simulink model "hexa_quaternion_observer_ANSFT"  (R2023a)
settings: Solver=ode1  StartTime=0.0  StopTime=5  FixedStep=0.01  RelTol=1e-3
undefined symbols (not defined in the file or in its folder): F, Light, MIL
libraries: dspsrcs4 x9, aerolibutil x8, sharedtransform x8, simulink x5, matrix_library x3, sharedutil x3, simulink_extras x3, robotcorelib x1, aerolibwind2 x1, uavutilslib x1
(part 1 of 2)
settings Model: Creator=adan  LastModifiedBy=adan

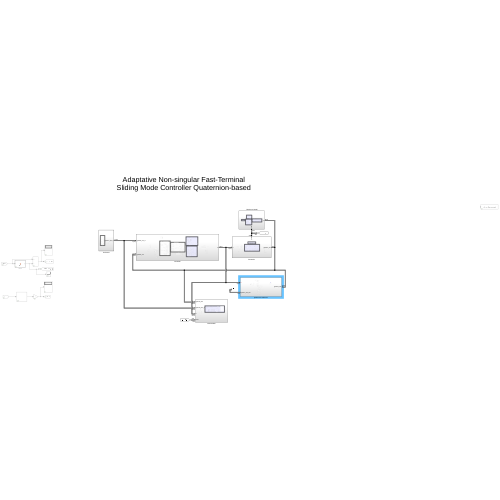
[thumbnail: Simulink's stored preview of the top-level diagram]
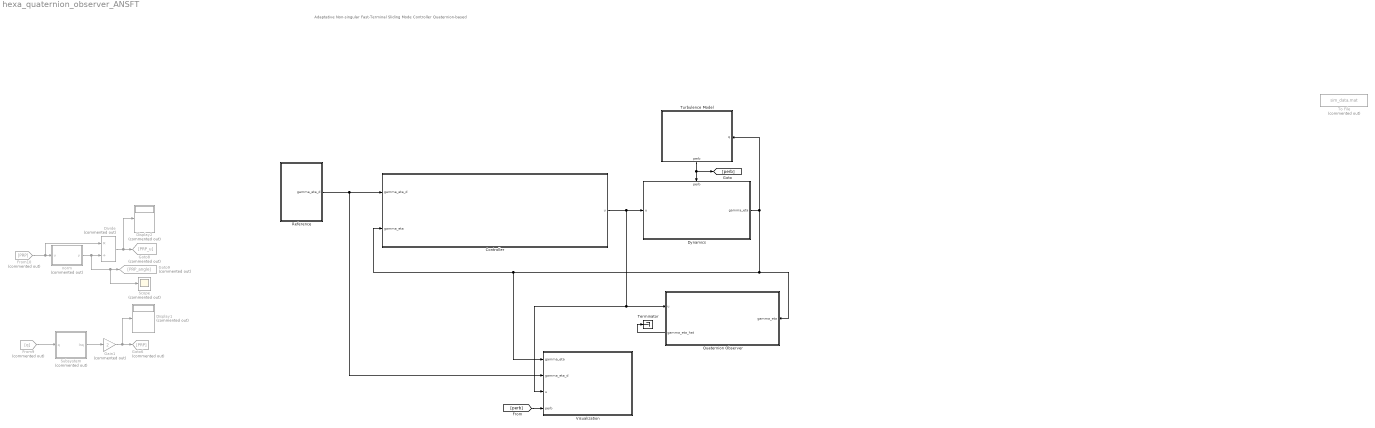
== system hexa_quaternion_observer_ANSFT ==
  note: Adaptative Non-singular Fast-Terminal Sliding Mode Controller Quaternion-based
  Controller : Subsystem
  Display1 : Display  Commented=on
  Display2 : Display  Commented=on
  Divide : Product  Commented=on  Inputs=*/
  Dynamics : Subsystem
      settings: PortSchema="{\"entries\":[{\"content\":{\"sides\":[{\"content\":{\"connectorIds\":[\"In1\"]},\"type\":\"ConnectorPlacement.EquallySpacedRectSide\",\"uuid\":\"7633f0a6-af79-48e6-9c86-d26739dbb2cd\"},{\"content\":{\"connectorIds\":[\"Out1\"],\"side\":\"RIGHT\"},\"type\":\"ConnectorPlacement.EquallySpacedRectSide\",\"uuid\":\"142aa0cc-a83e-43d8-8343-5180a7a0e227\"},{\"content\":{\"connectorIds\":[\"In2\"],\"side\":\"TOP\"},\"type\":\"ConnectorPlacement.EquallySpacedRectSide\",\"uuid\":\"a56720e4-09a6-4924-9ad2-7923d5a06f98\"}]},\"type\":\"ConnectorPlacement.EquallySpacedConnector\",\"uuid\":\"53d234f7-5315-4b90-bf85-0e64865b94b3\"}],\"packageUris\":[\"http://schema.mathworks.com/mf0/Connector/R2020b\"],\"version\":\"1.0\"}"
  From10 : From  Commented=on  GotoTag=PRP
  From9 : From  Commented=on  GotoTag=q
  Gain1 : Gain  Commented=on  Gain=2
  Goto6 : Goto  Commented=on  GotoTag=PRP
  Goto8 : Goto  Commented=on  GotoTag=PRP_u
  Goto9 : Goto  Commented=on  GotoTag=PRP_angle
  Quaternion Observer : Subsystem
      settings: PortSchema="{\"entries\":[{\"content\":{\"sides\":[{\"content\":{\"connectorIds\":[\"In1\"]},\"type\":\"ConnectorPlacement.EquallySpacedRectSide\",\"uuid\":\"43dabb6c-5b7b-4e74-9fbb-877aa2e7320c\"},{\"content\":{\"connectorIds\":[\"In2\",\"Out1\"],\"side\":\"RIGHT\"},\"type\":\"ConnectorPlacement.EquallySpacedRectSide\",\"uuid\":\"9ed47776-94ef-4325-8624-b198cf9ddeb6\"},{\"content\":{\"side\":\"TOP\"},\"type\":\"ConnectorPlacement.EquallySpacedRectSide\",\"uuid\":\"b1e3d92d-3c8b-4698-8faf-48c27cfda7a8\"}]},\"type\":\"ConnectorPlacement.EquallySpacedConnector\",\"uuid\":\"a3be4682-1c06-4ed6-a307-3a935f166e03\"}],\"packageUris\":[\"http://schema.mathworks.com/mf0/Connector/R2020b\"],\"version\":\"1.0\"}"
  Reference : Subsystem
  Scope : Scope  Commented=on
  Subsystem : Subsystem  Commented=on
  Terminator : Terminator
  To File : ToFile  Commented=on  Filename=sim_data.mat  MatrixName=out
  Turbulence Model : Subsystem
      settings: PortSchema="{\"entries\":[{\"content\":{\"sides\":[{\"content\":{},\"type\":\"ConnectorPlacement.EquallySpacedRectSide\",\"uuid\":\"1a11629b-61d3-4a8e-8df8-8509e014e579\"},{\"content\":{\"connectorIds\":[\"In1\"],\"side\":\"RIGHT\"},\"type\":\"ConnectorPlacement.EquallySpacedRectSide\",\"uuid\":\"4b15c564-9714-4da5-9436-a08c0d95800f\"},{\"content\":{\"side\":\"TOP\"},\"type\":\"ConnectorPlacement.EquallySpacedRectSide\",\"uuid\":\"dd21b825-2def-4360-b27b-b8c6f475bfab\"},{\"content\":{\"connectorIds\":[\"Out1\"],\"side\":\"BOTTOM\"},\"type\":\"ConnectorPlacement.EquallySpacedRectSide\",\"uuid\":\"594b79ea-4a45-43b1-b592-64a34d0135fb\"}]},\"type\":\"ConnectorPlacement.EquallySpacedConnector\",\"uuid\":\"4c6e67eb-825c-4dd0-a48b-2afa68ae74f5\"}],\"packageUris\":[\"http://schema.mathworks.com/mf0/Connector/R2020b\"],\"version\":\"1.0\"}"
  Visualization : Subsystem
  norm : MATLAB Function  Commented=on  TreatAsAtomicUnit=on
  wires:
  From9/1 -> Subsystem/1(q)
  Subsystem/1(lnq) -> Gain1/1
  Gain1/1 -> Display1/1, Goto6/1
  From10/1 -> norm/1(u), Divide/1
  norm/1(y) -> Scope/1, Goto9/1, Divide/2
  Divide/1 -> Goto8/1, Display2/1
  Reference/1(gamma_eta_d) -> Controller/1(gamma_eta_d), Visualization/2(gamma_eta_d)
  Controller/1(u) -> Quaternion Observer/2(u), Visualization/3(u), Dynamics/1(u)
  Dynamics/1(gamma_eta) -> Turbulence Model/1(q), Quaternion Observer/1(gamma_eta), Visualization/1(gamma_eta), Controller/2(gamma_eta)
  Turbulence Model/1(perb) -> [perb], Dynamics/2(perb)
  Quaternion Observer/1(gamma_eta_hat) -> Terminator/1
  [perb] -> Visualization/4(perb)

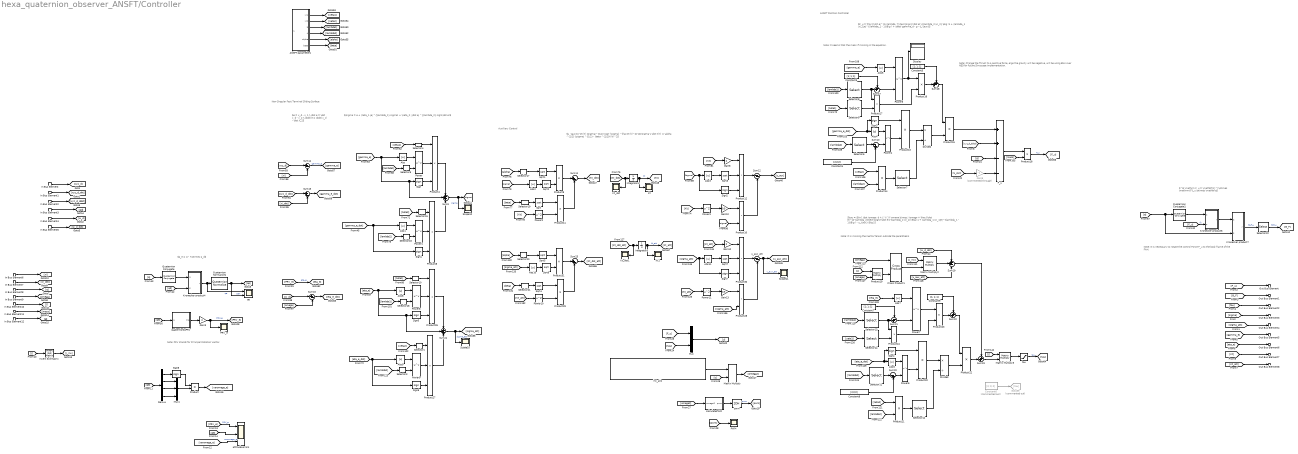
== system hexa_quaternion_observer_ANSFT/Controller ==
  note: $q_e = q^ *\otimes q_d$
  note: Non-Singular Fast Terminal Sliding Surface
  note: $\sigma = e + \zeta_1 |e| ^{\lambda_1} sign(e) + \zeta_2 | \dot e| ^{\lambda_2} sign(\dot e)$
  note: $F_u = \frac{|\dot e|^{2-\lambda_2}\text{sign}(\dot e)}{\lambda_2 \xi_2} \Big (1 + \lambda_1 \xi_1|e|^{\lambda_1 - 1}\Big ) + \ddot \gamma_d - g - u_{aux}$
  note: $\tau = \Big [ \dot \omega_d + J^{-1} \omega \times J \omega + \frac{|\dot e|^{2-\lambda_2}\text{sign}(\dot e)}{\lambda_2 \xi_2} \Big (1 + \lambda_1 \xi_1|e|^{\lambda_1 - 1}\Big ) - u_{aux} \Big ]$
  note: ANSFT Position Controller
  note: Note: It seems that the mass if missing in
      | the equation.
  note: $e = x_d - x_1 \\ \dot e = \dot x_d - x_2 \\ \ddot e = \ddot x_d - \dot x_2$
  note: Note: It is missing the Inertia Tensor outside
      | the parenthesis
  note: Auxiliary Control
  note: $u_{aux}=-2K(t) |\sigma|^{1/2} sign (\sigma) - \frac{K(t)^2}{2}\sigma \\ \dot K(t) = \alpha ^{1/2} |\sigma| ^{1/2} - \beta ^{1/2}K(t)^2$
  note: Note: Change the Thrust to a positive force, ergo the gravity will be negative,
      | will be using ENU over NED for future Simscape implementation.
  note: $^B \mathrm F_u = \mathbf{q}^*\otimes \mathrm{F}_u \otimes \mathbf q$
  note: Note: It is necessary to rotate the control Force F_u
      | to the body frame of the FAH.
  note: Note: PRV stands for Principal Rotation
      | Vector.
  In Bus Element : Inport  PortName=gamma_eta_d  Element=xyz_d
  In Bus Element1 : Inport  PortName=gamma_eta_d  Element=xyz_d_dot
  In Bus Element2 : Inport  PortName=gamma_eta_d  Element=xyz_d_ddot
  In Bus Element3 : Inport  PortName=gamma_eta_d  Element=qd
  In Bus Element4 : Inport  PortName=gamma_eta_d  Element=w_d
  In Bus Element5 : Inport  PortName=gamma_eta_d  Element=w_d_dot
  In Bus Element6 : Inport  Port=2  PortName=gamma_eta  Element=x
  In Bus Element7 : Inport  Port=2  PortName=gamma_eta  Element=x_dot
  In Bus Element8 : Inport  Port=2  PortName=gamma_eta  Element=q
  In Bus Element9 : Inport  Port=2  PortName=gamma_eta  Element=omega
  In Bus Element10 : Inport  Port=2  PortName=gamma_eta  Element=J
  In Bus Element11 : Inport  Port=2  PortName=gamma_eta  Element=m
  In Bus Element12 : Inport  Port=2  PortName=gamma_eta  Element=g
  ANSFT parameters : MATLAB Function  TreatAsAtomicUnit=on
  Abs{,1..11} (12 alike) : Abs  SaturateOnIntegerOverflow=off
  Constant{3,5,7,9} (4 alike) : Constant  Value=[1; 1; 1]
  Constant4 : Constant  Value=[2;2;2]
  Constant6 : Constant  Commented=on  Value=[0; 0; 0]
  Constant8 : Constant  Value=[2;2;2]
  Cross Product1 : matrix_library/Cross Product
  Demux : Demux
  Display : Display
  Divide2 : Product  Inputs=*/
  Divide3 : Product  Inputs=*/
  F_u : Sum  Inputs=++--
  Gain10 : Gain  Gain=0.5
  Gain12 : Gain  Gain=2
  Gain13 : Gain  Gain=0.5
  Gain3 : Gain  Gain=2
  Gain6 : Gain  Commented=through  Gain=-1
  Gain8 : Gain  Gain=2
  Goto59 : Goto  Commented=on  GotoTag=tau
  Integrator4 : Integrator  InitialCondition=[0;0;0]
  Integrator5 : Integrator  InitialCondition=[0;0;0]
  Invert 3x3 Matrix : aerolibutil/Invert  3x3 Matrix
  Kronecker product4 : Subsystem
  Kronecker product6 : Subsystem
  Kronecker product7 : Subsystem
  Kt : Scope
  Kt1 : Scope
  Kt_dot : Scope
  Kt_dot1 : Scope
  Matrix Multiply : Product  Multiplication=Matrix(*)
  Matrix Multiply2 : Product  Multiplication=Matrix(*)
  Matrix Multiply5 : Product  Multiplication=Matrix(*)
  Mux : Mux  Inputs=2
  Mux1 : Mux  Inputs=3
  PRV_e : Scope
  PWM : Scope
  Power{,1,4..9} (8 alike) : Math  Operator=pow
  Power{2..3,10..11} (4 alike) : Math  Operator=square
  Product{,9..11,13..18,20..24,28..29,31} (18 alike) : Product
  Product{4,8,12,26..27,30} (6 alike) : Product  Inputs=3
  Product19 : Product  Multiplication=Matrix(*)
  Quaternion Conjugate : aerolibutil/Quaternion Conjugate
  Quaternion Conjugate1 : aerolibutil/Quaternion Conjugate
  Quaternion Normalize1 : sharedutil/Quaternion Normalize  aMode=aMode
  Scope10 : Scope
  Scope11 : Scope
  Scope12 : Scope
  Selector{1,3,10..14,18,20..21} (10 alike) : Selector  InputPortWidth=6  IndexOptions=Index vector (dialog)  Indices=[4:6]  OutputSizes=1
  Selector{4..9,15..17,19} (10 alike) : Selector  InputPortWidth=6  IndexOptions=Index vector (dialog)  Indices=[1:3]  OutputSizes=1
  Selector22 : Selector  InputPortWidth=4  IndexOptions=Index vector (dialog)  Indices=[2:4]  OutputSizes=1
  Sign{,1..8} (9 alike) : Signum
  Sqrt{,1..7} (8 alike) : Sqrt
  Sum10 : Sum  Inputs=|-+
  Sum{11,14..16,25} (5 alike) : Sum  Inputs=|+-
  Sum12 : Sum  Inputs=|--
  Sum17 : Sum  Inputs=-+|
  Sum18 : Sum  Inputs=++|
  Sum19 : Sum  Inputs=++-
  Sum20 : Sum  Inputs=|-+
  Sum21 : Sum  Inputs=-+|
  Sum22 : Sum  Inputs=++|
  Sum23 : Sum  Inputs=++|
  Sum24 : Sum  Inputs=+++
  Sum9 : Sum  Inputs=+++
  attitude errors : Scope  NumInputPorts=3
  calculatePWM : MATLAB Function  TreatAsAtomicUnit=on
  inv_allo : Constant  Value=|
      | [-0.6436    0.3716    0.1352    0.8869   -0.5120    1.1817;
      |             0.6436    0.3716    0.1352    0.8869    0.5120   -1.1817;
      |             -0.0000   -0.7431    0.1352    0.0000    1.0241    1.1817;
      |             -0.6436    0.3716    0.1352   -0.8869    0.5120   -1.1817;
      |             0.6436    0.3716    0.1352   -0.8869   -0.5120    1.1817;
      |             0.0000   -0.7431    0.1352   -0.0000   -1.0241   -1.1817;] * 1.0e+05;
  pwm : ZeroOrderHold  SampleTime=-1
  qe : Scope  NumInputPorts=2
  quaterniontoPRV : Subsystem
  tau : Saturate
  u_aux_att : Sum  Inputs=|--
  Out Bus Element : Outport  PortName=u  Element=F_u
  Out Bus Element1 : Outport  PortName=u  Element=B-F_u
  Out Bus Element2 : Outport  PortName=u  Element=tau
  Out Bus Element3 : Outport  PortName=u  Element=sigma
  Out Bus Element4 : Outport  PortName=u  Element=sigma_att
  Out Bus Element5 : Outport  PortName=u  Element=gamma_e
  Out Bus Element6 : Outport  PortName=u  Element=eta_e
  Out Bus Element7 : Outport  PortName=u  Element=Kt
  Out Bus Element8 : Outport  PortName=u  Element=Kt_att
  wires:
  Product19/1 -> Cross Product1/2
  [tau] -> Mux/2
  [u_aux_att] -> Sum19/3
  Abs8/1 -> Power8/1
  Sum18/1 -> Product15/1
  Mux/1 -> [u]
  [omega2] -> calculatePWM/1(omega2)
  [xi] -> Sum14/2
  [xi_dot] -> Sum15/2
  Sqrt7/1 -> Product30/2
  Selector10/1 -> Product26/1
  Divide3/1 -> Product22/2
  Matrix Multiply/1 -> [omega2]
  [lambda2] -> Product14/2
  [w_d_dot] -> Sum19/1
  Product22/1 -> Sum23/2
  Sqrt2/1 -> Product9/2
  Sum25/1 -> [Kt_dot_att]
  [mass] -> Product18/2
  inv_allo/1 -> Matrix Multiply/1
  Abs3/1 -> Sqrt3/1
  [xyz_d_ddot] -> F_u/2
  [u] -> Matrix Multiply/2
  Selector21/1 -> Sqrt4/1
  [zeta1] -> Selector9/1
  [F_u] -> Mux/1
  [J] -> Matrix Multiply5/1
  Product26/1 -> Sum24/1
  Gain12/1 -> Product30/1
  [lambda2] -> Selector11/1
  [sigma] -> Product10/2
  Product15/1 -> F_u/1
  Sign2/1 -> Product12/3
  Product8/1 -> Sum9/3
  Abs6/1 -> Power6/1
  Product16/1 -> Sum18/2
  Sqrt/1 -> Product11/1
  [Kt_dot] -> Kt_dot/1, Integrator4/1
  [lambda1] -> Selector8/1
  Abs4/1 -> Power4/1
  Integrator5/1 -> Kt1/1, [Kt_att]  "Kt_att"
  F_u/1 -> Product18/1
  Product11/1 -> Sum11/2
  Product18/1 -> [F_u]  "F_u"
  Abs5/1 -> Power5/1
  tau/1 -> [tau]  "tau"
  [Kt_att] -> Power10/1
  [Kt] -> Power2/1
  Product10/1 -> Sum12/2
  Gain13/1 -> Product28/1
  Selector13/1 -> Product24/1, Sum21/2
  Sum10/1 -> Power4/2
  Sum19/1 -> Sum23/1
  Selector11/1 -> Sum20/1
  Product12/1 -> Sum12/1
  [eta_e_dot] -> Abs9/1, Sign6/1
  Matrix Multiply5/1 -> tau/1
  Selector4/1 -> Product4/1
  Power/1 -> Product4/2
  [lambda2] -> Selector3/1
  Selector12/1 -> Divide3/2
  Selector18/1 -> Power8/2
  Power10/1 -> Product29/2
  Gain6/1 -> F_u/4
  Sum22/1 -> Product22/1
  [w_d] -> Sum16/1
  Product9/1 -> Sum11/1
  Sqrt6/1 -> Product31/2
  Gain8/1 -> Product12/1
  Selector9/1 -> Product17/2
  Selector14/1 -> Product24/2
  [zeta2] -> Product21/1
  Sqrt5/1 -> Product31/1
  [pwm] -> PWM/1
  Sign5/1 -> Product26/3
  Sign/1 -> Product4/3
  [zeta1] -> Selector14/1
  Constant8/1 -> Sum20/2
  Abs7/1 -> Power7/1
  Power5/1 -> Display/1, Product16/1
  [sigma_att] -> Abs11/1, Sign7/1
  Product23/1 -> Sum22/2
  Selector7/1 -> Divide2/2
  Abs10/1 -> Sqrt6/1
  [eta_e] -> Abs7/1
  Sign6/1 -> Product27/3
  Selector6/1 -> Sum10/1
  Constant3/1 -> Sum17/1
  [xyz_d_dot] -> Sum15/1
  Sum15/1 -> [gamma_e_dot]
  [zeta2] -> Product14/1
  [xyz_d] -> Sum14/1
  [lambda2] -> Product21/2
  Sum12/1 -> [u_aux]
  Sqrt3/1 -> Product12/2
  Sum24/1 -> Scope10/1, [sigma_att]  "sigma_att"
  [lambda2] -> Selector16/1
  Cross Product1/1 -> Matrix Multiply2/2
  Product24/1 -> Product23/2
  [alpha] -> Selector20/1
  [sigma] -> Abs2/1
  Selector16/1 -> Power1/2
  [eta_e_dot] -> Sign4/1, Abs6/1
  Selector8/1 -> Product17/1, Sum17/2
  Selector1/1 -> Product27/1
  [beta] -> Selector21/1
  Constant7/1 -> Sum21/1
  Integrator4/1 -> Kt/1, [Kt]  "Kt"
  Sum23/1 -> Matrix Multiply5/2
  Power8/1 -> Product26/2
  [Kt] -> Power3/1
  [Kt] -> Gain8/1
  Product30/1 -> u_aux_att/1
  [gamma_e_dot] -> Sign1/1, Abs1/1
  Selector3/1 -> Power9/2
  [J_inv] -> Matrix Multiply2/1
  [u_aux] -> Gain6/1
  [alpha] -> Selector17/1
  Selector19/1 -> Sqrt/1
  Divide2/1 -> Product15/2
  [eta_e] -> Sum24/2, Sign5/1, Abs8/1
  [gamma_e] -> Sum9/2, Sign/1, Abs/1
  Constant9/1 -> Sum22/1
  [omega] -> Sum16/2
  [J] -> Product19/1
  Sign7/1 -> Product30/3
  Sqrt4/1 -> Product29/1
  [Kt_att] -> Power11/1
  Abs2/1 -> Sqrt2/1
  Power9/1 -> Product27/2
  calculatePWM/1(pwm) -> pwm/1
  [zeta2] -> Selector15/1
  Selector17/1 -> Sqrt1/1
  Product20/1 -> Divide3/1
  Product13/1 -> Divide2/1
  [g] -> F_u/3
  [PRV_e] -> [eta_e]  "eta_e"
  Sum21/1 -> Power7/2
  Power7/1 -> Product23/1
  Constant5/1 -> Sum18/1
  Sum14/1 -> [gamma_e]  "gamma_e"
  [Kt_att] -> Gain12/1
  Sum20/1 -> Power6/2
  [lambda2] -> Selector6/1
  Selector20/1 -> Sqrt5/1
  [sigma] -> Sign2/1, Abs3/1
  [sigma_att] -> Product28/2
  Sum11/1 -> [Kt_dot]
  Abs11/1 -> Sqrt7/1
  [zeta2] -> Selector1/1
  [gamma_e] -> Abs5/1
  Sign1/1 -> Product8/3
  Product17/1 -> Product16/2
  Selector15/1 -> Product8/1
  Power2/1 -> Product11/2
  Abs1/1 -> Power1/1
  Constant6/1 -> Goto59/1
  Power11/1 -> Gain13/1
  [lambda1] -> Selector18/1
  Matrix Multiply2/1 -> Sum19/2
  u_aux_att/1 -> Scope11/1, [u_aux_att]  "u_aux_att"
  pwm/1 -> [pwm]  "pwm"
  Sign4/1 -> Product20/1
  Power1/1 -> Product8/2
  [omega] -> Cross Product1/1
  Product31/1 -> Sum25/1
  Power4/1 -> Product13/2
  Constant4/1 -> Sum10/2
  Product28/1 -> u_aux_att/2
  Product4/1 -> Sum9/1
  Product14/1 -> Selector7/1
  [gamma_e_dot] -> Sign3/1, Abs4/1
  Selector5/1 -> Power/2
  Product27/1 -> Sum24/3
  Abs9/1 -> Power9/1
  Sum17/1 -> Power5/2
  Sum16/1 -> [eta_e_dot]
  Product29/1 -> Sum25/2
  Abs/1 -> Power/1
  [zeta1] -> Selector4/1
  [sigma_att] -> Abs10/1
  Power3/1 -> Gain10/1
  Sum9/1 -> Scope12/1, [sigma]  "sigma"
  Product21/1 -> Selector12/1
  [zeta1] -> Selector10/1
  [beta] -> Selector19/1
  Gain10/1 -> Product10/1
  [omega] -> Product19/2
  Sign3/1 -> Product13/1
  [lambda1] -> Selector5/1
  [lambda1] -> Selector13/1
  Power6/1 -> Product20/2
  [Kt_dot_att] -> Kt_dot1/1, Integrator5/1
  Sqrt1/1 -> Product9/1
  ANSFT parameters/4(lambda2) -> [lambda2]
  ANSFT parameters/6(beta) -> [beta]
  ANSFT parameters/3(lambda1) -> [lambda1]
  ANSFT parameters/2(xi2) -> [zeta2]
  ANSFT parameters/1(xi1) -> [zeta1]
  ANSFT parameters/5(alpha) -> [alpha]
  Kronecker product6/1(r) -> Kronecker product7/1(q)
  Quaternion Conjugate1/1 -> Kronecker product6/1(q)
  [q] -> Kronecker product7/2(p), Quaternion Conjugate1/1
  Selector22/1 -> [B_F]  "B-F_u"
  Kronecker product7/1(r) -> Selector22/1  "B_F_u"
  [F_u] -> Kronecker product6/2(p)  "fu"
  In Bus Element/1 -> [xyz_d]
  In Bus Element1/1 -> [xyz_d_dot]
  In Bus Element4/1 -> [w_d]
  In Bus Element3/1 -> [qd]
  In Bus Element2/1 -> [xyz_d_ddot]
  In Bus Element5/1 -> [w_d_dot]
  quaterniontoPRV/1(lnq) -> Gain3/1
  [qd] -> Kronecker product4/2(p)
  [q] -> Quaternion Conjugate/1
  Quaternion Conjugate/1 -> Kronecker product4/1(q)
  Kronecker product4/1(r) -> qe/1, Quaternion Normalize1/1  "qe"
  Quaternion Normalize1/1 -> qe/2, [qe]  "qen"
  Gain3/1 -> PRV_e/1, [PRV_e]  "PRV_e"
  [qe] -> quaterniontoPRV/1(q)
  [F_u] -> Out Bus Element/1
  [B_F] -> Out Bus Element1/1
  [tau] -> Out Bus Element2/1
  [sigma] -> Out Bus Element3/1
  [sigma_att] -> Out Bus Element4/1
  [gamma_e] -> Out Bus Element5/1
  [eta_e] -> Out Bus Element6/1
  [Kt] -> Out Bus Element7/1
  [Kt_att] -> Out Bus Element8/1
  In Bus Element8/1 -> [q]
  In Bus Element9/1 -> [omega]
  In Bus Element7/1 -> [xi_dot]
  In Bus Element6/1 -> [xi]
  In Bus Element12/1 -> [g]
  In Bus Element11/1 -> [mass]
  In Bus Element10/1 -> [J]
  [J] -> Invert 3x3 Matrix/1
  Invert 3x3 Matrix/1 -> [J_inv]
  [qe] -> Demux/1
  Demux/1 -> Sign8/1
  Demux/3 -> Mux1/2
  Demux/2 -> Mux1/1
  Demux/4 -> Mux1/3
  Mux1/1 -> Product/2
  Sign8/1 -> Product/1
  Product/1 -> [varomega_e]
  [qe] -> attitude errors/2
  [PRV_e] -> attitude errors/1  "PRV_e"
  [varomega_e] -> attitude errors/3  "varomega_e"

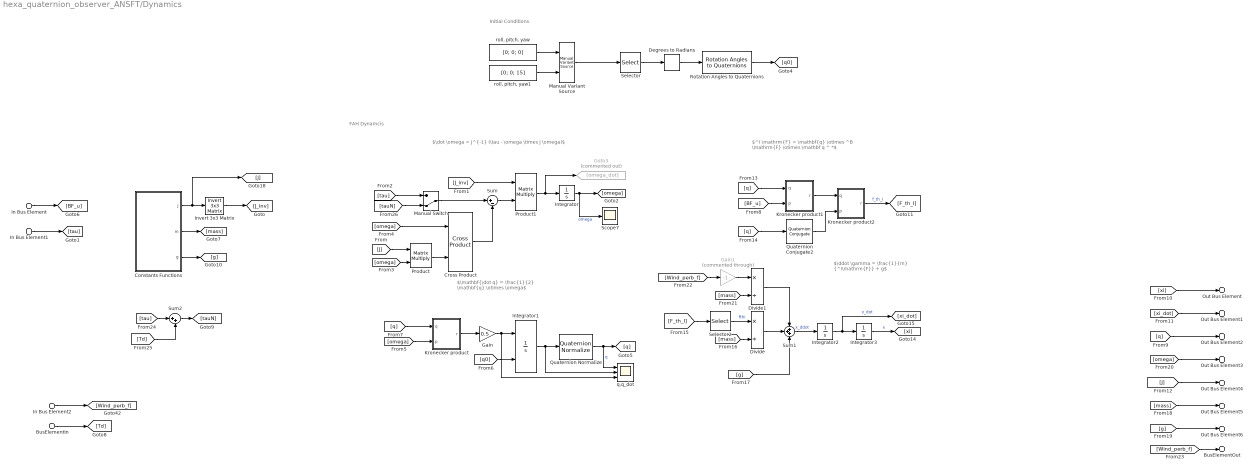
== system hexa_quaternion_observer_ANSFT/Dynamics ==
  note: $^I \mathrm{F} = \mathbf{q} \otimes ^B \mathrm{F} \otimes \mathbf q ^ *$
  note: FAH Dynamcis
  note: $\ddot \gamma = \frac{1}{m} {^I\mathrm{F}} + g$
  note: $\mathbf{\dot q} = \frac{1}{2} \mathbf{q} \otimes \omega$
  note: $\dot \omega = J^{-1} (\tau - \omega \times J \omega)$
  note: Initial Conditions
  In Bus Element : Inport  PortName=u  Element=B-F_u
  In Bus Element1 : Inport  PortName=u  Element=tau
  In Bus Element2 : Inport  Port=2  PortName=perb  Element=perb
  BusElementIn : Inport  Port=2  PortName=perb  Element=Td
  Constants Functions : MATLAB Function  TreatAsAtomicUnit=on
  Cross Product : matrix_library/Cross Product
  Degrees to Radians : simulink_extras/Transformations/Degrees to Radians
  Divide : Product  Inputs=*/
  Divide1 : Product  Inputs=*/
  Gain : Gain  Gain=0.5
  Gain1 : Gain  Commented=through  Gain=-1
  Goto3 : Goto  Commented=on  GotoTag=omega_dot
  Integrator : Integrator  InitialCondition=[0; 0; 0]
  Integrator1 : Integrator  InitialConditionSource=external
  Integrator2 : Integrator  InitialCondition=[0; 0; 0]
  Integrator3 : Integrator  InitialCondition=[0; 0; 0]
  Invert 3x3 Matrix : aerolibutil/Invert  3x3 Matrix
  Kronecker product : Subsystem
      mask Display: image('$imagefile'); % Use "Edit Image" on toolstrip to change.
  Kronecker product1 : Subsystem
  Kronecker product2 : Subsystem
  Manual Variant Source : simulink/Signal Routing/Manual Variant Source  NumChoices=2  LabelModeActiveChoice=V_1
  Manual Switch : ManualSwitch  CurrentSetting=0
  Product : Product  Multiplication=Matrix(*)
  Product1 : Product  Multiplication=Matrix(*)
  Quaternion Conjugate2 : aerolibutil/Quaternion Conjugate
  Quaternion Normalize : sharedutil/Quaternion Normalize  aMode=aMode
  Rotation Angles to Quaternions : sharedtransform/Rotation Angles to Quaternions  rotationOrder=ZYX  aMode=aMode
  Scope7 : Scope
  Selector : Selector  InputPortWidth=3  IndexOptions=Index vector (dialog)  Indices=[3 2 1]  OutputSizes=1
  Selector2 : Selector  InputPortWidth=4  IndexOptions=Index vector (dialog)  Indices=[2:4]  OutputSizes=1
  Sum : Sum  Inputs=|+-
  Sum1 : Sum  Inputs=+++
  Sum2 : Sum  Inputs=|++
  q,q_dot : Scope  NumInputPorts=3
  "roll, pitch, yaw" : Constant  Value=[0; 0; 0]
  "roll, pitch, yaw1" : Constant  Value=[0; 0; 15]
  Out Bus Element : Outport  PortName=gamma_eta  Element=x
  Out Bus Element1 : Outport  PortName=gamma_eta  Element=x_dot
  Out Bus Element2 : Outport  PortName=gamma_eta  Element=q
  Out Bus Element3 : Outport  PortName=gamma_eta  Element=omega
  Out Bus Element4 : Outport  PortName=gamma_eta  Element=J
  Out Bus Element5 : Outport  PortName=gamma_eta  Element=m
  Out Bus Element6 : Outport  PortName=gamma_eta  Element=g
  BusElementOut : Outport  PortName=gamma_eta  Element=perb
  wires:
  Constants Functions/2(m) -> [mass]
  [BF_u] -> Kronecker product1/2(p)
  [q0] -> Integrator1/2
  Integrator1/1 -> q,q_dot/2, Quaternion Normalize/1
  Kronecker product1/1(r) -> Kronecker product2/1(q)
  [J] -> Product/1
  Product/1 -> Cross Product/2
  [q] -> Kronecker product1/1(q)
  Manual Variant Source/1 -> Selector/1
  Sum/1 -> Product1/2
  [F_th_I] -> Selector2/1
  Quaternion Conjugate2/1 -> Kronecker product2/2(p)
  Kronecker product/1(r) -> Gain/1
  "roll, pitch, yaw1"/1 -> Manual Variant Source/2
  Gain/1 -> q,q_dot/3, Integrator1/1
  Integrator3/1 -> [xi]  "x"
  "roll, pitch, yaw"/1 -> Manual Variant Source/1
  Integrator2/1 -> [xi_dot], Integrator3/1  "x_dot"
  [q] -> Quaternion Conjugate2/1
  Constants Functions/1(J) -> [J], Invert 3x3 Matrix/1
  [omega] -> Cross Product/1
  Selector/1 -> Degrees to Radians/1
  [omega] -> Kronecker product/2(p)
  [q] -> Kronecker product/1(q)
  Product1/1 -> Goto3/1, Integrator/1
  Invert 3x3 Matrix/1 -> [J_inv]
  Constants Functions/3(g) -> [g]
  Sum1/1 -> Integrator2/1  "x_ddot"
  Integrator/1 -> Scope7/1, [omega]  "omega"
  Cross Product/1 -> Sum/2
  Degrees to Radians/1 -> Rotation Angles to Quaternions/1
  [omega] -> Product/2
  [J_inv] -> Product1/1
  [tau] -> Manual Switch/1
  Rotation Angles to Quaternions/1 -> [q0]
  Kronecker product2/1(r) -> [F_th_I]  "f_th_I"
  Quaternion Normalize/1 -> q,q_dot/1, [q]  "q"
  Selector2/1 -> Divide/1  "fthi"
  [mass] -> Divide/2
  In Bus Element/1 -> [BF_u]
  In Bus Element1/1 -> [tau]
  [xi] -> Out Bus Element/1
  [xi_dot] -> Out Bus Element1/1
  [q] -> Out Bus Element2/1
  [omega] -> Out Bus Element3/1
  [J] -> Out Bus Element4/1
  [mass] -> Out Bus Element5/1
  [g] -> Out Bus Element6/1
  Divide/1 -> Sum1/2
  [g] -> Sum1/3
  [mass] -> Divide1/2
  Divide1/1 -> Sum1/1
  In Bus Element2/1 -> [Wind_perb_f]
  [Wind_perb_f] -> Gain1/1
  [Wind_perb_f] -> BusElementOut/1
  Gain1/1 -> Divide1/1
  BusElementIn/1 -> [Td]
  [tau] -> Sum2/1
  [Td] -> Sum2/2
  Sum2/1 -> [tauN]
  Manual Switch/1 -> Sum/1
  [tauN] -> Manual Switch/2

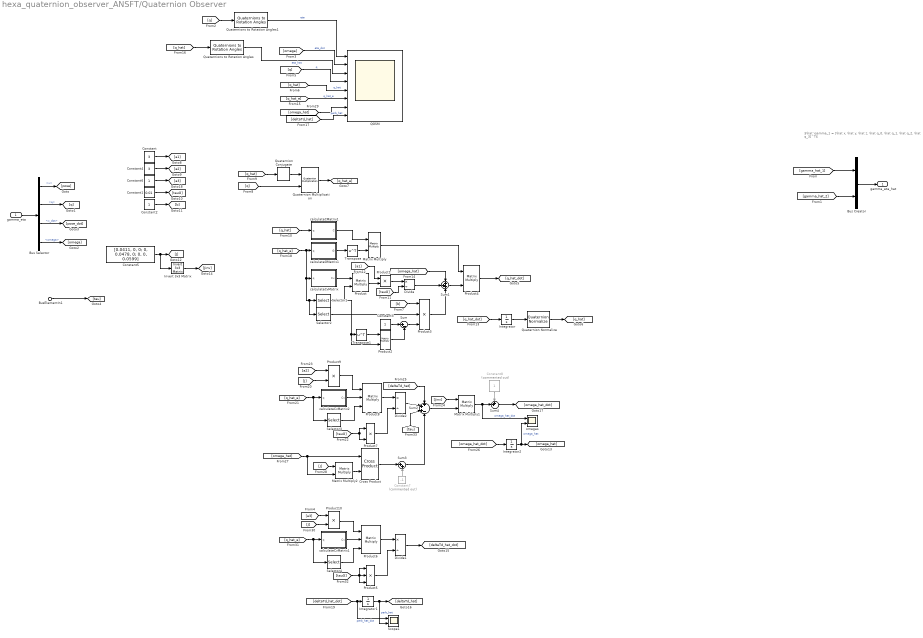
== system hexa_quaternion_observer_ANSFT/Quaternion Observer ==
  note: $\hat \gamma_1 = [\hat x, \hat y, \hat z, \hat q_0, \hat q_1, \hat q_2, \hat q_3]^T$
  gamma_eta : Inport
  BusElementIn1 : Inport  Port=2  PortName=u  Element=tau
  Bus Creator : BusCreator  Inputs=2
  Bus Selector : BusSelector  OutputSignals=x,q,x_dot,omega
  Constant : Constant  Value=3
  Constant1 : Constant  Value=0.01
  Constant2 : Constant
  Constant3 : Constant
  Constant4 : Constant  Value=3
  Constant5 : Constant  Value=[0.0411, 0, 0; 0, 0.0478, 0; 0, 0, 0.0599]
  Constant6 : Constant
  Constant7 : Constant  Commented=on  Value=-1
  Constant8 : Constant  Commented=on
  Cross Product : matrix_library/Cross Product
  Divide : Product  Inputs=*/
  Divide1 : Product  Inputs=*/
  Divide2 : Product  Inputs=*/
  Integrator : Integrator  InitialCondition=[1; 0; 0; 0]
  Integrator1 : Integrator  InitialCondition=[0; 0; 0]
  Integrator2 : Integrator  InitialCondition=[0; 0; 0]
  Invert 3x3 Matrix : aerolibutil/Invert  3x3 Matrix
  Matrix Multiply : Product  Multiplication=Matrix(*)
  Matrix Multiply1 : Product  Multiplication=Matrix(*)
  Matrix Multiply2 : Product  Multiplication=Matrix(*)
  Product : Product  Multiplication=Matrix(*)
  Product{1,7,9..10} (4 alike) : Product
  Product2 : Product  Multiplication=Matrix(*)
  Product3 : Product  Inputs=3
  Product4 : Product  Multiplication=Matrix(*)
  Product5 : Product  Inputs=3
  Product6 : Product  Inputs=3  Multiplication=Matrix(*)
  Product8 : Product  Inputs=3  Multiplication=Matrix(*)
  QOSM : Scope  NumInputPorts=8
  Quaternion Conjugate : aerolibutil/Quaternion Conjugate
  Quaternion Multiplication : aerolibutil/Quaternion Multiplication
  Quaternion Normalize : sharedutil/Quaternion Normalize  aMode=aMode
  Quaternions to Rotation Angles : sharedtransform/Quaternions to Rotation Angles  rotationOrder=XYZ  aMode=aMode
  Quaternions to Rotation Angles1 : sharedtransform/Quaternions to Rotation Angles  rotationOrder=XYZ  aMode=aMode
  Scope1 : Scope  NumInputPorts=2
  Selector1 : Selector  InputPortWidth=4  IndexOptions=Index vector (dialog)  Indices=[2:4]  OutputSizes=1
  Selector2 : Selector  InputPortWidth=4  IndexOptions=Index vector (dialog)  Indices=[1]  OutputSizes=1
  Selector3 : Selector  InputPortWidth=4  IndexOptions=Index vector (dialog)  Indices=[2:4]  OutputSizes=1
  Selector4 : Selector  InputPortWidth=4  IndexOptions=Index vector (dialog)  Indices=[2:4]  OutputSizes=1
  Sum : Sum  Inputs=|+-
  Sum1 : Sum  Inputs=+++
  Sum2 : Sum  Inputs=+++-
  Sum3 : Sum  Inputs=|++
  Sum4 : Sum  Inputs=++|
  Transpose : Math  Operator=transpose
  Transpose1 : Math  Operator=transpose
  calculateCMatrix1 : MATLAB Function  TreatAsAtomicUnit=on
  calculateCvMatrix : MATLAB Function  TreatAsAtomicUnit=on
  calculateCvMatrix1 : MATLAB Function  TreatAsAtomicUnit=on
  calculateCvMatrix2 : MATLAB Function  TreatAsAtomicUnit=on
  calculateGMatrix1 : MATLAB Function  TreatAsAtomicUnit=on
  omegas : Scope  NumInputPorts=2
  gamma_eta_hat : Outport
  wires:
  gamma_eta/1 -> Bus Selector/1
  Bus Selector/1 -> [pose]  "<x>"
  Bus Creator/1 -> gamma_eta_hat/1
  [gamma_hat_2] -> Bus Creator/2
  [gamma_hat_1] -> Bus Creator/1
  Bus Selector/4 -> [omega]  "<omega>"
  Bus Selector/3 -> [pose_dot]  "<x_dot>"
  Bus Selector/2 -> [q]  "<q>"
  BusElementIn1/1 -> [tau]
  [omega_hat] -> QOSM/7
  Quaternions to Rotation Angles1/1 -> QOSM/1  "eta"
  [q_hat] -> Quaternions to Rotation Angles/1
  [q] -> QOSM/4  "q"
  [omega] -> QOSM/2  "eta_dot"
  [q_hat_e] -> QOSM/6  "q_hat_e"
  Quaternions to Rotation Angles/1 -> QOSM/3  "eta_hat"
  [deltaTd_hat] -> QOSM/8  "perb_hat"
  [q_hat] -> QOSM/5  "q_hat"
  Constant1/1 -> [tauG]
  Constant2/1 -> [b]
  Constant/1 -> [a1]
  Constant5/1 -> Invert 3x3 Matrix/1, [J]
  Invert 3x3 Matrix/1 -> [Jinv]
  Quaternion Conjugate/1 -> Quaternion Multiplication/1
  [q] -> Quaternion Multiplication/2
  [q_hat] -> Quaternion Conjugate/1
  Quaternion Multiplication/1 -> [q_hat_e]
  Divide/1 -> Sum1/2
  [q_hat_e] -> Selector2/1, Selector1/1, calculateCvMatrix/1(q), calculateGMatrix1/1(q)
  [q_hat_dot] -> Integrator/1
  Product3/1 -> Sum1/3
  Matrix Multiply/1 -> Product4/1
  Sum1/1 -> Product4/2
  Selector2/1 -> Product3/2
  Product2/1 -> Sum/2
  Quaternion Normalize/1 -> [q_hat]
  [omega_hat] -> Sum1/1
  Constant3/1 -> Sum/1
  Integrator/1 -> Quaternion Normalize/1
  Product1/1 -> Divide/1
  [q_hat] -> calculateCMatrix1/1(q)
  calculateCMatrix1/1(C) -> Matrix Multiply/1
  calculateCvMatrix/1(Cv) -> Product/1
  Selector1/1 -> Product2/2, Transpose1/1, Product/2
  Sum/1 -> Product3/3
  [tauG] -> Divide/2
  calculateGMatrix1/1(G) -> Transpose/1
  Product4/1 -> [q_hat_dot]
  Transpose/1 -> Matrix Multiply/2
  [a1] -> Product1/1
  Transpose1/1 -> Product2/1
  calculateCvMatrix2/1(Cv) -> Product8/2
  Sum2/1 -> Matrix Multiply1/2
  [a2] -> Product9/1
  [tauG] -> Product7/2, Product7/1
  [Jinv] -> Matrix Multiply1/1
  [omega_hat] -> Cross Product/1, Matrix Multiply2/2
  [q_hat_e] -> Selector3/1, calculateCvMatrix2/1(q)
  Product8/1 -> Divide2/1
  Matrix Multiply2/1 -> Cross Product/2
  [J] -> Matrix Multiply2/1
  Matrix Multiply1/1 -> Sum4/2, omegas/1  "omega_hat_dot"
  Selector3/1 -> Product8/3
  [omega_hat_dot] -> Integrator2/1
  Product7/1 -> Divide2/2
  [J] -> Product9/2
  Product9/1 -> Product8/1
  Integrator2/1 -> omegas/2, [omega_hat]  "omega_hat"
  [deltaTd_hat] -> Sum2/1
  Divide2/1 -> Sum2/2
  Product6/1 -> Divide1/1
  Selector4/1 -> Product6/3
  [tauG] -> Product5/3, Product5/1, Product5/2
  calculateCvMatrix1/1(Cv) -> Product6/2
  [deltaTd_hat_dot] -> Scope1/1, Integrator1/1  "perb_hat_dot"
  [J] -> Product10/2
  Integrator1/1 -> Scope1/2, [deltaTd_hat]  "perb_hat"
  [q_hat_e] -> Selector4/1, calculateCvMatrix1/1(q)
  Product5/1 -> Divide1/2
  Divide1/1 -> [deltaTd_hat_dot]
  [q] -> Quaternions to Rotation Angles1/1
  Product/1 -> Product1/2
  Constant4/1 -> [a2]
  Constant6/1 -> [a3]
  [a3] -> Product10/1
  Product10/1 -> Product6/1
  [tau] -> Sum2/3
  [b] -> Product3/1
  Cross Product/1 -> Sum3/1
  Sum3/1 -> Sum2/4
  Constant7/1 -> Sum3/2
  Sum4/1 -> [omega_hat_dot]
  Constant8/1 -> Sum4/1

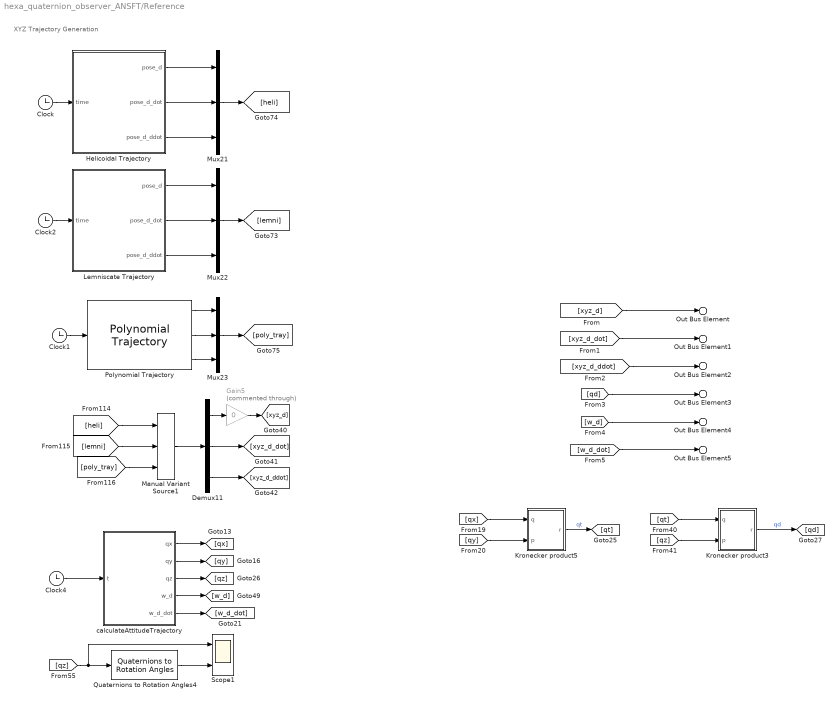
== system hexa_quaternion_observer_ANSFT/Reference ==
  note: XYZ Trajectory Generation
  Clock{,1..2,4} (4 alike) : Clock
  Demux11 : Demux  Outputs=3
  Gain5 : Gain  Commented=through  Gain=0
  Helicoidal Trajectory : MATLAB Function  TreatAsAtomicUnit=on
  Kronecker product3 : Subsystem
  Kronecker product5 : Subsystem
  Lemniscate Trajectory : MATLAB Function  TreatAsAtomicUnit=on
  Manual Variant Source1 : simulink/Signal Routing/Manual Variant Source  NumChoices=3  LabelModeActiveChoice=V_3
  Mux21 : Mux  Inputs=3
  Mux22 : Mux  Inputs=3
  Mux23 : Mux  Inputs=3
  Polynomial Trajectory : robotcorelib/Polynomial Trajectory  WaypointSource=Internal  Waypoints=zeros(3, 6)  TimePoints=[ 0, 12, 24, 36, 48, 60]  TimeInterval=[ 1, 4 ]  Method=Cubic Polynomial  ParameterSource=Internal  VelocityBoundaryCondition=zeros( 3, 6)  AccelerationBoundaryCondition=zeros( 2, 5 )  SimulateUsing=Interpreted execution
  Quaternions to Rotation Angles4 : sharedtransform/Quaternions to Rotation Angles  rotationOrder=ZYX  aMode=aMode
  Scope1 : Scope  NumInputPorts=2
  calculateAttitudeTrajectory : MATLAB Function  TreatAsAtomicUnit=on
  Out Bus Element : Outport  PortName=gamma_eta_d  Element=xyz_d
  Out Bus Element1 : Outport  PortName=gamma_eta_d  Element=xyz_d_dot
  Out Bus Element2 : Outport  PortName=gamma_eta_d  Element=xyz_d_ddot
  Out Bus Element3 : Outport  PortName=gamma_eta_d  Element=qd
  Out Bus Element4 : Outport  PortName=gamma_eta_d  Element=w_d
  Out Bus Element5 : Outport  PortName=gamma_eta_d  Element=w_d_dot
  wires:
  Mux23/1 -> [poly_tray]
  [poly_tray] -> Manual Variant Source1/3
  [qz] -> Scope1/1, Quaternions to Rotation Angles4/1
  Clock/1 -> Helicoidal Trajectory/1(time)
  Demux11/2 -> [xyz_d_dot]
  Lemniscate Trajectory/3(pose_d_ddot) -> Mux22/3
  Quaternions to Rotation Angles4/1 -> Scope1/2
  Demux11/1 -> Gain5/1
  Manual Variant Source1/1 -> Demux11/1
  calculateAttitudeTrajectory/3(qz) -> [qz]
  Lemniscate Trajectory/2(pose_d_dot) -> Mux22/2
  Polynomial Trajectory/2 -> Mux23/2
  Helicoidal Trajectory/3(pose_d_ddot) -> Mux21/3
  Mux21/1 -> [heli]
  calculateAttitudeTrajectory/4(w_d) -> [w_d]
  Lemniscate Trajectory/1(pose_d) -> Mux22/1
  Helicoidal Trajectory/1(pose_d) -> Mux21/1
  Demux11/3 -> [xyz_d_ddot]
  [heli] -> Manual Variant Source1/1
  calculateAttitudeTrajectory/1(qx) -> [qx]
  [lemni] -> Manual Variant Source1/2
  Gain5/1 -> [xyz_d]
  calculateAttitudeTrajectory/5(w_d_dot) -> [w_d_dot]
  Clock4/1 -> calculateAttitudeTrajectory/1(t)
  Clock2/1 -> Lemniscate Trajectory/1(time)
  Polynomial Trajectory/1 -> Mux23/1
  calculateAttitudeTrajectory/2(qy) -> [qy]
  Mux22/1 -> [lemni]
  Clock1/1 -> Polynomial Trajectory/1
  Polynomial Trajectory/3 -> Mux23/3
  Helicoidal Trajectory/2(pose_d_dot) -> Mux21/2
  [qy] -> Kronecker product5/2(p)
  [qx] -> Kronecker product5/1(q)
  [qz] -> Kronecker product3/2(p)
  Kronecker product5/1(r) -> [qt]  "qt"
  Kronecker product3/1(r) -> [qd]  "qd"
  [qt] -> Kronecker product3/1(q)
  [xyz_d_ddot] -> Out Bus Element2/1
  [xyz_d_dot] -> Out Bus Element1/1
  [xyz_d] -> Out Bus Element/1
  [w_d_dot] -> Out Bus Element5/1
  [w_d] -> Out Bus Element4/1
  [qd] -> Out Bus Element3/1

== system hexa_quaternion_observer_ANSFT/Subsystem ==
  q : Inport
  MATLAB Function : MATLAB Function  TreatAsAtomicUnit=on
  lnq : Outport
  wires:
  MATLAB Function/1(lnq) -> lnq/1
  q/1 -> MATLAB Function/1(q)

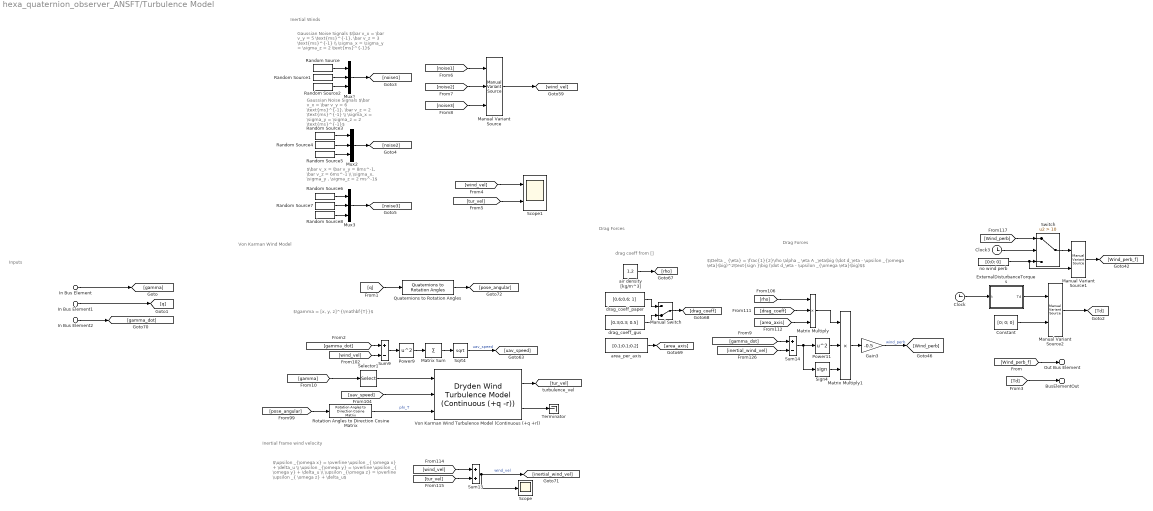
== system hexa_quaternion_observer_ANSFT/Turbulence Model ==
  note: Von Karman Wind Model
  note: Drag Forces
  note: Inputs
  note: Inertial Winds
  note: Gaussian Noise Signals
      | $\bar v_x = \bar v_y = 6 \text{ms}^{-1}, \bar v_z = 2 \text{ms}^{-1} \\ \sigma_x = \sigma_y = \sigma_z = 2 \text{ms}^{-1}$
  note: Gaussian Noise Signals
      | $\bar v_x = \bar v_y = 5 \text{ms}^{-1}, \bar v_z = 3 \text{ms}^{-1} \\ \sigma_x = \sigma_y = \sigma_z = 2 \text{ms}^{-1}$
  note: $\Delta _ {\eta} = \frac{1}{2}\rho \alpha _ \eta A _\eta\big (\dot d_\eta - \upsilon _{\omega \eta}\big)^2\text{sign }\big (\dot d_\eta - \upsilon _{\omega \eta}\big)$$
  note: drag coeff from []
  note: $\upsilon _{\omega x} = \overline \upsilon _{ \omega x} + \delta_u \\ \upsilon _{\omega y} = \overline \upsilon _{ \omega y} + \delta_u \\ \upsilon _{\omega z} = \overline \upsilon _{ \omega z} + \delta_u$
  note: $\gamma = [x, y, z]^{\mathbf{T}}$
  note: Drag Forces
  note: Inertial frame wind velocity
  note: $\bar v_x = \bar v_y = 8ms^-1, \bar v_z = 6ms^-1 \\ \sigma_x, \sigma_y , \sigma_z = 2 ms^-1$
  In Bus Element : Inport  PortName=q  Element=x
  In Bus Element1 : Inport  PortName=q  Element=q
  In Bus Element2 : Inport  PortName=q  Element=x_dot
  Clock : Clock
  Clock3 : Clock
  Constant : Constant  Value=[0; 0; 0]
  ExternalDisturbanceTorques : MATLAB Function  TreatAsAtomicUnit=on
  Gain3 : Gain  Gain=-0.5
  Manual Variant Source : simulink/Signal Routing/Manual Variant Source  NumChoices=3  LabelModeActiveChoice=V_1
  Manual Variant Source1 : simulink/Signal Routing/Manual Variant Source  NumChoices=2  LabelModeActiveChoice=V_2
  Manual Variant Source2 : simulink/Signal Routing/Manual Variant Source  NumChoices=2  LabelModeActiveChoice=V_2
  Manual Switch : ManualSwitch  CurrentSetting=0
  Matrix Sum : Sum  Inputs=+
  Matrix Multiply : Product  Inputs=3
  Matrix Multiply1 : Product  Inputs=3
  Mux1 : Mux  Inputs=3
  Mux2 : Mux  Inputs=3
  Mux3 : Mux  Inputs=3
  Power11 : Math  Operator=square
  Power9 : Math  Operator=square
  Quaternions to Rotation Angles : sharedtransform/Quaternions to Rotation Angles  rotationOrder=XYZ  aMode=aMode
  Random Source : dspsrcs4/Random Source  SrcType=Gaussian  NormMethod=Ziggurat  CltLength=12  MinVal=0  MaxVal=1  MeanVal=5  VarVal=2  RepMode=Not repeatable  rawSeed=1  IsInherit=off  SampMode=Discrete  SampTime=1  SampFrame=1  DataType=Double  OutComplex=Real  OutputFrames=off
  Random Source1 : dspsrcs4/Random Source  SrcType=Gaussian  NormMethod=Ziggurat  CltLength=12  MinVal=0  MaxVal=1  MeanVal=5  VarVal=2  RepMode=Not repeatable  rawSeed=1  IsInherit=off  SampMode=Discrete  SampTime=1  SampFrame=1  DataType=Double  OutComplex=Real  OutputFrames=off
  Random Source2 : dspsrcs4/Random Source  SrcType=Gaussian  NormMethod=Ziggurat  CltLength=12  MinVal=0  MaxVal=1  MeanVal=3  VarVal=2  RepMode=Not repeatable  rawSeed=1  IsInherit=off  SampMode=Discrete  SampTime=1  SampFrame=1  DataType=Double  OutComplex=Real  OutputFrames=off
  Random Source3 : dspsrcs4/Random Source  SrcType=Gaussian  NormMethod=Ziggurat  CltLength=12  MinVal=0  MaxVal=1  MeanVal=6  VarVal=2  RepMode=Not repeatable  rawSeed=1  IsInherit=off  SampMode=Discrete  SampTime=1  SampFrame=1  DataType=Double  OutComplex=Real  OutputFrames=off
  Random Source4 : dspsrcs4/Random Source  SrcType=Gaussian  NormMethod=Ziggurat  CltLength=12  MinVal=0  MaxVal=1  MeanVal=6  VarVal=2  RepMode=Not repeatable  rawSeed=1  IsInherit=off  SampMode=Discrete  SampTime=1  SampFrame=1  DataType=Double  OutComplex=Real  OutputFrames=off
  Random Source5 : dspsrcs4/Random Source  SrcType=Gaussian  NormMethod=Ziggurat  CltLength=12  MinVal=0  MaxVal=1  MeanVal=2  VarVal=2  RepMode=Not repeatable  rawSeed=1  IsInherit=off  SampMode=Discrete  SampTime=1  SampFrame=1  DataType=Double  OutComplex=Real  OutputFrames=off
  Random Source6 : dspsrcs4/Random Source  SrcType=Gaussian  NormMethod=Ziggurat  CltLength=12  MinVal=0  MaxVal=1  MeanVal=8  VarVal=2  RepMode=Not repeatable  rawSeed=1  IsInherit=off  SampMode=Discrete  SampTime=1  SampFrame=1  DataType=Double  OutComplex=Real  OutputFrames=off
  Random Source7 : dspsrcs4/Random Source  SrcType=Gaussian  NormMethod=Ziggurat  CltLength=12  MinVal=0  MaxVal=1  MeanVal=8  VarVal=2  RepMode=Not repeatable  rawSeed=1  IsInherit=off  SampMode=Discrete  SampTime=1  SampFrame=1  DataType=Double  OutComplex=Real  OutputFrames=off
  Random Source8 : dspsrcs4/Random Source  SrcType=Gaussian  NormMethod=Ziggurat  CltLength=12  MinVal=0  MaxVal=1  MeanVal=6  VarVal=2  RepMode=Not repeatable  rawSeed=1  IsInherit=off  SampMode=Discrete  SampTime=1  SampFrame=1  DataType=Double  OutComplex=Real  OutputFrames=off
  Rotation Angles to Direction Cosine Matrix : sharedtransform/Rotation Angles to Direction Cosine Matrix  rotationOrder=XYZ  aMode=aMode
  Scope : Scope
  Scope1 : Scope  NumInputPorts=2
  Selector1 : Selector  InputPortWidth=3  IndexOptions=Index vector (dialog)  Indices=[3]  OutputSizes=1
  Sign4 : Signum
  Sqrt4 : Sqrt
  Sum13 : Sum
  Sum14 : Sum  Inputs=+-
  Sum9 : Sum  Inputs=+-
  Switch : Switch  Criteria=u2 > Threshold  Threshold=10  SaturateOnIntegerOverflow=off  InputSameDT=off
  Terminator : Terminator
  Von Karman Wind Turbulence Model (Continuous (+q +r)) : aerolibwind2/Dryden Wind Turbulence Model  (Continuous (+q -r))  units=Metric (MKS)  spec=MIL-F-8785C  model=Continuous Von Karman (+q -r)  W20=15.43  Wdeg=0  TurbProb=10^-2 - Light  L_high=762  Wingspan=10  ts=0.1  Seed=[23341 23342 23343 23344]  T_on=on
      settings: LibrarySourceBlock=|
      | aerolibwind2/Von Karman Wind Turbulence Model
      | (Continuous (+q +r))
  air density [kg/m^3] : Constant  Value=1.2
  area_per_axis : Constant  Value=[0.1;0.1;0.2]
  drag_coeff_gus : Constant  Value=[0.3;0.3; 0.5]
  drag_coeff_paper : Constant  Value=[0.6;0.6; 1]
  no wind perb : Constant  Value=[0;0; 0]
  Out Bus Element : Outport  PortName=perb  Element=perb
  BusElementOut : Outport  PortName=perb  Element=Td
  wires:
  [rho] -> Matrix Multiply/1
  Manual Switch/1 -> [drag_coeff]
  Power11/1 -> Matrix Multiply1/2
  Von Karman Wind Turbulence Model (Continuous (+q +r))/1 -> [tur_vel]
  Rotation Angles to Direction Cosine Matrix/1 -> Von Karman Wind Turbulence Model (Continuous (+q +r))/3  "phi_T"
  drag_coeff_paper/1 -> Manual Switch/1
  Matrix Sum/1 -> Sqrt4/1
  Gain3/1 -> [Wind_perb]  "wind_perb"
  Matrix Multiply/1 -> Matrix Multiply1/1
  Quaternions to Rotation Angles/1 -> [pose_angular]
  Sum9/1 -> Power9/1
  no wind perb/1 -> Manual Variant Source1/2, Switch/3
  Clock3/1 -> Switch/2
  Sum14/1 -> Sign4/1, Power11/1
  [area_axis] -> Matrix Multiply/3
  Von Karman Wind Turbulence Model (Continuous (+q +r))/2 -> Terminator/1
  [uav_speed] -> Von Karman Wind Turbulence Model (Continuous (+q +r))/2
  [drag_coeff] -> Matrix Multiply/2
  air density [kg/m^3]/1 -> [rho]
  area_per_axis/1 -> [area_axis]
  [pose_angular] -> Rotation Angles to Direction Cosine Matrix/1
  drag_coeff_gus/1 -> Manual Switch/2
  Sum13/1 -> Scope/1, [inertial_wind_vel]  "wind_vel"
  [gamma_dot] -> Sum9/1
  [tur_vel] -> Sum13/2
  Selector1/1 -> Von Karman Wind Turbulence Model (Continuous (+q +r))/1
  [gamma_dot] -> Sum14/1
  [wind_vel] -> Sum9/2
  [Wind_perb] -> Switch/1
  [wind_vel] -> Sum13/1
  Sqrt4/1 -> [uav_speed]  "uav_speed"
  Sign4/1 -> Matrix Multiply1/3
  Power9/1 -> Matrix Sum/1
  Matrix Multiply1/1 -> Gain3/1
  [inertial_wind_vel] -> Sum14/2
  [Wind_perb_f] -> Out Bus Element/1
  In Bus Element2/1 -> [gamma_dot]
  In Bus Element1/1 -> [q]
  [q] -> Quaternions to Rotation Angles/1
  Switch/1 -> Manual Variant Source1/1
  [wind_vel] -> Scope1/1
  [tur_vel] -> Scope1/2
  Random Source/1 -> Mux1/1
  Random Source1/1 -> Mux1/2
  Random Source2/1 -> Mux1/3
  Mux1/1 -> [noise1]
  Random Source4/1 -> Mux2/2
  Random Source5/1 -> Mux2/3
  Random Source3/1 -> Mux2/1
  Mux2/1 -> [noise2]
  Manual Variant Source/1 -> [wind_vel]
  [noise2] -> Manual Variant Source/2
  [noise3] -> Manual Variant Source/3
  [noise1] -> Manual Variant Source/1
  Random Source7/1 -> Mux3/2
  Random Source6/1 -> Mux3/1
  Random Source8/1 -> Mux3/3
  Mux3/1 -> [noise3]
  In Bus Element/1 -> [gamma]
  [gamma] -> Selector1/1
  Manual Variant Source1/1 -> [Wind_perb_f]
  Clock/1 -> ExternalDisturbanceTorques/1(t)
  ExternalDisturbanceTorques/1(Td) -> Manual Variant Source2/1
  [Td] -> BusElementOut/1
  Constant/1 -> Manual Variant Source2/2
  Manual Variant Source2/1 -> [Td]

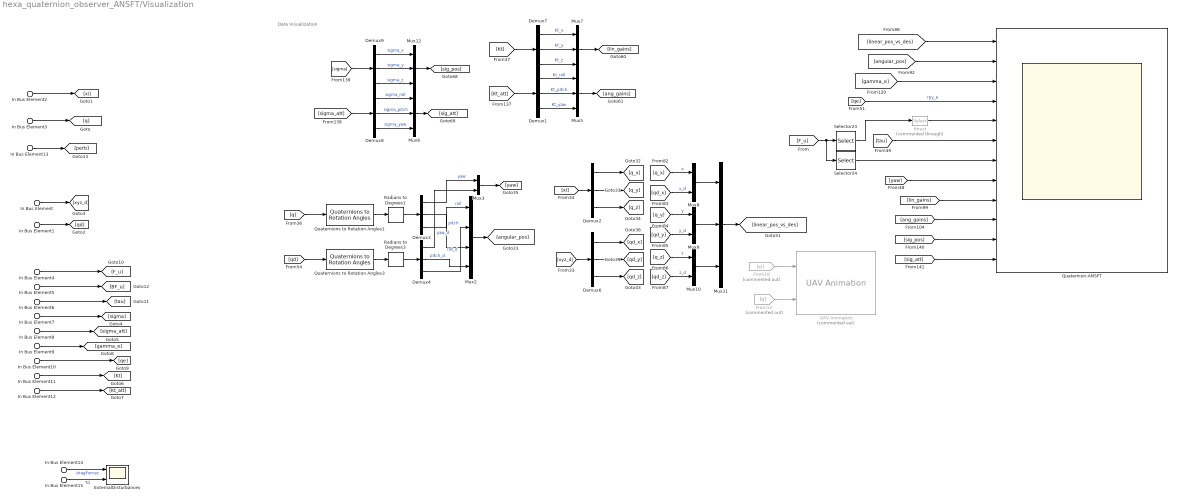
== system hexa_quaternion_observer_ANSFT/Visualization ==
  note: Data Visualization
  In Bus Element2 : Inport  PortName=gamma_eta  Element=x
  In Bus Element3 : Inport  PortName=gamma_eta  Element=q
  In Bus Element13 : Inport  PortName=gamma_eta  Element=perb
  In Bus Element : Inport  Port=2  PortName=gamma_eta_d  Element=xyz_d
  In Bus Element1 : Inport  Port=2  PortName=gamma_eta_d  Element=qd
  In Bus Element4 : Inport  Port=3  PortName=u  Element=F_u
  In Bus Element5 : Inport  Port=3  PortName=u  Element=B-F_u
  In Bus Element6 : Inport  Port=3  PortName=u  Element=tau
  In Bus Element7 : Inport  Port=3  PortName=u  Element=sigma
  In Bus Element8 : Inport  Port=3  PortName=u  Element=sigma_att
  In Bus Element9 : Inport  Port=3  PortName=u  Element=gamma_e
  In Bus Element10 : Inport  Port=3  PortName=u  Element=eta_e
  In Bus Element11 : Inport  Port=3  PortName=u  Element=Kt
  In Bus Element12 : Inport  Port=3  PortName=u  Element=Kt_att
  In Bus Element14 : Inport  Port=4  PortName=perb  Element=perb
  In Bus Element15 : Inport  Port=4  PortName=perb  Element=Td
  Demux{1..4,6..9} (8 alike) : Demux  Outputs=3
  ExternalDisturbances : Scope  NumInputPorts=2
  From12 : From  Commented=on  GotoTag=q
  From18 : From  Commented=on  GotoTag=xi
  Mux{3,8..10} (4 alike) : Mux  Inputs=2
  Mux{5..7,11..12} (5 alike) : Mux  Inputs=3
  Mux2 : Mux
  Quaternion-ANSFT : Scope  NumInputPorts=12
  Quaternions to Rotation Angles1 : sharedtransform/Quaternions to Rotation Angles  rotationOrder=ZYX  aMode=aMode
  Quaternions to Rotation Angles3 : sharedtransform/Quaternions to Rotation Angles  rotationOrder=ZYX  aMode=aMode
  Radians to Degrees1 : simulink_extras/Transformations/Radians to Degrees
  Radians to Degrees3 : simulink_extras/Transformations/Radians to Degrees
  Selector23 : Selector  InputPortWidth=3  IndexOptions=Index vector (dialog)  Indices=[3]  OutputSizes=1
  Selector24 : Selector  InputPortWidth=3  IndexOptions=Index vector (dialog)  Indices=[1:2]  OutputSizes=1
  UAV Animation : uavutilslib/UAV Animation  Commented=on  UAVType=Multirotor  UAVSize=1  InertialZDirection=Down  SampleTime=-1
  thrust : Selector  Commented=through  InputPortWidth=3  IndexOptions=Index vector (dialog)  Indices=[3]  OutputSizes=1
  wires:
  [sigma_att] -> Demux8/1
  Radians to Degrees1/1 -> Demux3/1
  Demux3/3 -> Mux2/1  "roll"
  [lin_gains] -> Quaternion-ANSFT/9
  Mux11/1 -> [linear_pos_vs_des]
  [qe] -> Quaternion-ANSFT/4  "rpy_e"
  Mux3/1 -> [yaw]
  Demux6/1 -> [qd_x]
  Demux9/2 -> Mux12/2  "sigma_y"
  [yaw] -> Quaternion-ANSFT/8
  Mux5/1 -> [ang_gains]
  Mux10/1 -> Mux11/3
  Demux1/1 -> Mux5/1  "Kt_roll"
  Demux7/3 -> Mux7/3  "Kt_z"
  From12/1 -> UAV Animation/2
  [q_z] -> Mux10/1  "z"
  [linear_pos_vs_des] -> Quaternion-ANSFT/1
  Quaternions to Rotation Angles1/1 -> Radians to Degrees1/1
  [Kt] -> Demux7/1
  Demux4/2 -> Mux2/4  "pitch_d"
  Demux7/1 -> Mux7/1  "Kt_x"
  [qd] -> Quaternions to Rotation Angles3/1
  [qd_x] -> Mux8/2  "x_d"
  Demux7/2 -> Mux7/2  "Kt_y"
  Mux7/1 -> [lin_gains]
  Demux8/3 -> Mux6/3  "sigma_yaw"
  Demux6/2 -> [qd_y]
  [xyz_d] -> Demux6/1
  [gamma_e] -> Quaternion-ANSFT/3
  [sig_att] -> Quaternion-ANSFT/12
  [F_u] -> Selector24/1, Selector23/1
  Demux4/1 -> Mux3/2  "yaw_d"
  Selector24/1 -> Quaternion-ANSFT/7
  [q_x] -> Mux8/1  "x"
  [ang_gains] -> Quaternion-ANSFT/10
  Demux1/3 -> Mux5/3  "Kt_yaw"
  Mux9/1 -> Mux11/2
  Selector23/1 -> thrust/1
  Demux2/3 -> [q_z]
  Mux8/1 -> Mux11/1
  Demux3/1 -> Mux3/1  "yaw"
  [sig_pos] -> Quaternion-ANSFT/11
  [tau] -> Quaternion-ANSFT/6
  From18/1 -> UAV Animation/1
  Quaternions to Rotation Angles3/1 -> Radians to Degrees3/1
  Demux6/3 -> [qd_z]
  [q] -> Quaternions to Rotation Angles1/1
  Radians to Degrees3/1 -> Demux4/1
  [qd_z] -> Mux10/2  "z_d"
  Demux1/2 -> Mux5/2  "Kt_pitch"
  [qd_y] -> Mux9/2  "y_d"
  thrust/1 -> Quaternion-ANSFT/5
  Mux12/1 -> [sig_pos]
  Mux6/1 -> [sig_att]
  Demux2/2 -> [q_y]
  [sigma] -> Demux9/1
  Demux9/3 -> Mux12/3  "sigma_z"
  [q_y] -> Mux9/1  "y"
  Demux8/2 -> Mux6/2  "sigma_pitch"
  Demux2/1 -> [q_x]
  [Kt_att] -> Demux1/1
  Demux3/2 -> Mux2/3  "pitch"
  Mux2/1 -> [angular_pos]
  Demux9/1 -> Mux12/1  "sigma_x"
  Demux8/1 -> Mux6/1  "sigma_roll"
  [xi] -> Demux2/1
  [angular_pos] -> Quaternion-ANSFT/2
  Demux4/3 -> Mux2/2  "roll_d"
  In Bus Element3/1 -> [q]
  In Bus Element2/1 -> [xi]
  In Bus Element1/1 -> [qd]
  In Bus Element/1 -> [xyz_d]
  In Bus Element6/1 -> [tau]
  In Bus Element7/1 -> [sigma]
  In Bus Element8/1 -> [sigma_att]
  In Bus Element9/1 -> [gamma_e]
  In Bus Element10/1 -> [qe]
  In Bus Element4/1 -> [F_u]
  In Bus Element5/1 -> [BF_u]
  In Bus Element11/1 -> [Kt]
  In Bus Element12/1 -> [Kt_att]
  In Bus Element13/1 -> [perb]
  In Bus Element14/1 -> ExternalDisturbances/1  "dragForces"
  In Bus Element15/1 -> ExternalDisturbances/2  "Td"

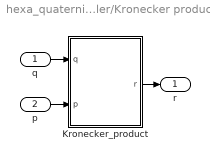
== system hexa_quaternion_observer_ANSFT/Controller/Kronecker product4 ==
  q : Inport
  p : Inport  Port=2
  Kronecker_product : MATLAB Function  TreatAsAtomicUnit=on
  r : Outport
  wires:
  q/1 -> Kronecker_product/1(q)
  p/1 -> Kronecker_product/2(p)
  Kronecker_product/1(r) -> r/1

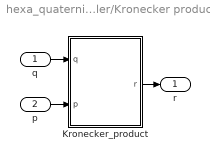
== system hexa_quaternion_observer_ANSFT/Controller/Kronecker product6 ==
  q : Inport
  p : Inport  Port=2
  Kronecker_product : MATLAB Function  TreatAsAtomicUnit=on
  r : Outport
  wires:
  q/1 -> Kronecker_product/1(q)
  p/1 -> Kronecker_product/2(p)
  Kronecker_product/1(r) -> r/1

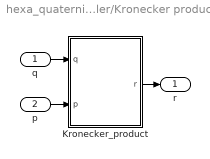
== system hexa_quaternion_observer_ANSFT/Controller/Kronecker product7 ==
  q : Inport
  p : Inport  Port=2
  Kronecker_product : MATLAB Function  TreatAsAtomicUnit=on
  r : Outport
  wires:
  q/1 -> Kronecker_product/1(q)
  p/1 -> Kronecker_product/2(p)
  Kronecker_product/1(r) -> r/1

== system hexa_quaternion_observer_ANSFT/Controller/quaterniontoPRV ==
  q : Inport
  MATLAB Function : MATLAB Function  TreatAsAtomicUnit=on
  lnq : Outport
  wires:
  MATLAB Function/1(lnq) -> lnq/1
  q/1 -> MATLAB Function/1(q)

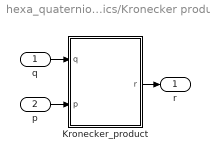
== system hexa_quaternion_observer_ANSFT/Dynamics/Kronecker product ==
  q : Inport
  p : Inport  Port=2
  Kronecker_product : MATLAB Function  TreatAsAtomicUnit=on
  r : Outport
  wires:
  q/1 -> Kronecker_product/1(q)
  p/1 -> Kronecker_product/2(p)
  Kronecker_product/1(r) -> r/1

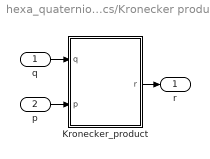
== system hexa_quaternion_observer_ANSFT/Dynamics/Kronecker product1 ==
  q : Inport
  p : Inport  Port=2
  Kronecker_product : MATLAB Function  TreatAsAtomicUnit=on
  r : Outport
  wires:
  q/1 -> Kronecker_product/1(q)
  p/1 -> Kronecker_product/2(p)
  Kronecker_product/1(r) -> r/1

== system hexa_quaternion_observer_ANSFT/Dynamics/Kronecker product2 ==
  q : Inport
  p : Inport  Port=2
  Kronecker_product : MATLAB Function  TreatAsAtomicUnit=on
  r : Outport
  wires:
  q/1 -> Kronecker_product/1(q)
  p/1 -> Kronecker_product/2(p)
  Kronecker_product/1(r) -> r/1

== system hexa_quaternion_observer_ANSFT/Reference/Kronecker product3 ==
  q : Inport
  p : Inport  Port=2
  Kronecker_product : MATLAB Function  TreatAsAtomicUnit=on
  r : Outport
  wires:
  q/1 -> Kronecker_product/1(q)
  p/1 -> Kronecker_product/2(p)
  Kronecker_product/1(r) -> r/1

== system hexa_quaternion_observer_ANSFT/Reference/Kronecker product5 ==
  q : Inport
  p : Inport  Port=2
  Kronecker_product : MATLAB Function  TreatAsAtomicUnit=on
  r : Outport
  wires:
  q/1 -> Kronecker_product/1(q)
  p/1 -> Kronecker_product/2(p)
  Kronecker_product/1(r) -> r/1

== matlab function hexa_quaternion_observer_ANSFT/Quaternion Observer/calculateCMatrix1 ==
  data: q input; C output
function C = fcn(q)

q0 = q(1);
q1 = q(2);
q2 = q(3);
q3 = q(4);

C = [-q1, -q2, -q3;
      q0, -q3, q2;
      q3, q0, -q1;
      -q2, q1, q0] * 0.5;

== matlab function hexa_quaternion_observer_ANSFT/Reference/Kronecker product3/Kronecker_product ==
  data: q input; r output size=[4 1]; p input
function r = fcn(q, p)

%{
    Function to describe in matrix math the Kronecker product between
    two quaternions
    
    r = p kronecker q
    %}

    len = length(p);

    if len == 3 && length(q) == 4
        p1 = [0; p];
        q0 = q(1);
        q1 = q(2);
        q2 = q(3);
        q3 = q(4);
        
        % skew symmetric matrix
        q_matrix = [q0, -q1, -q2, -q3;
                  q1, q0, -q3, q2;
                  q2, q3, q0, -q1;
                  q3, -q2, q1, q0];
        
        r = q_matrix * p1;

    elseif len == 4
        q0 = q(1);
        q1 = q(2);
        q2 = q(3);
        q3 = q(4);
        
        % skew symmetric matrix
        q_matrix = [q0, -q1, -q2, -q3;
                  q1, q0, -q3, q2;
                  q2, q3, q0, -q1;
                  q3, -q2, q1, q0];
        
        r = q_matrix * p;

    else
        error('Quaternions dimensions do not match')
    end

== matlab function hexa_quaternion_observer_ANSFT/Controller/quaterniontoPRV/MATLAB Function ==
  data: q input; lnq output size=[3 1]
function lnq = fcn(q)

if length(q) == 4
    q0 = q(1);
    q_vec = [q(2); q(3); q(4)];

    if norm(q_vec) == 0
        lnq = [0; 0; 0];
    else
        % q0 = real(q0);
        lnq = (q_vec / (norm(q_vec)) ) * acos(q0);
    end
else
    error('Input must be a vector 4 by 1 (Quaternion)')
end
